simulink model "Stateflow_Eventi"  (R2023b)
settings: Solver=VariableStepAuto  StartTime=0.0  StopTime=inf  RelTol=1e-3
settings Model: Creator=sabat  LastModifiedBy=sabat
settings SolverCC: AlgebraicLoopSolver=TrustRegion
settings OptimizationCC: DefaultParameterBehavior=Inlined  EnhancedBackFolding=on  PassReuseOutputArgsAs=Individual arguments  ZeroExternalMemoryAtStartup=off  ZeroInternalMemoryAtStartup=off  OptimizeBlockOrder=speed  DifferentSizesBufferReuse=on  OptimizationCustomize=off  EfficientTunableParamExpr=on
settings DebuggingCC: ParameterTunabilityLossMsg=error
settings SFSimCC: MATLABDynamicMemAlloc=off
settings RTWCC: Description=Embedded Coder  SystemTargetFile=ert.tlc  TemplateMakefile=ert_default_tmf
settings CodeAppCC: ForceParamTrailComments=on  IgnoreCustomStorageClasses=off  OperatorAnnotations=on  SimulinkDataObjDesc=on  SFDataObjDesc=on  InsertBlockDesc=on
settings ERTTargetCC: TargetLangStandard=C99 (ISO)  GenerateSampleERTMain=on  InlinedParameterPlacement=NonHierarchical  ERTCustomFileTemplate=example_file_process.tlc

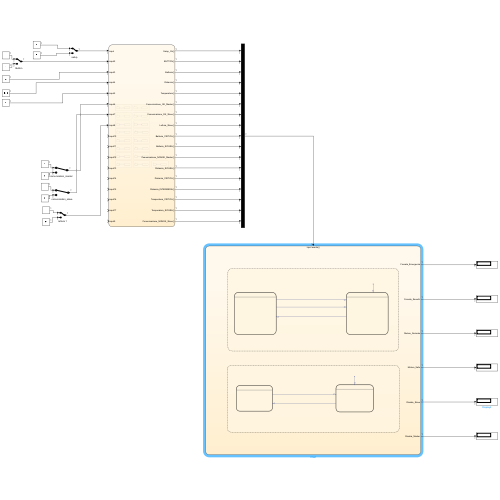
[thumbnail: Simulink's stored preview of the top-level diagram]
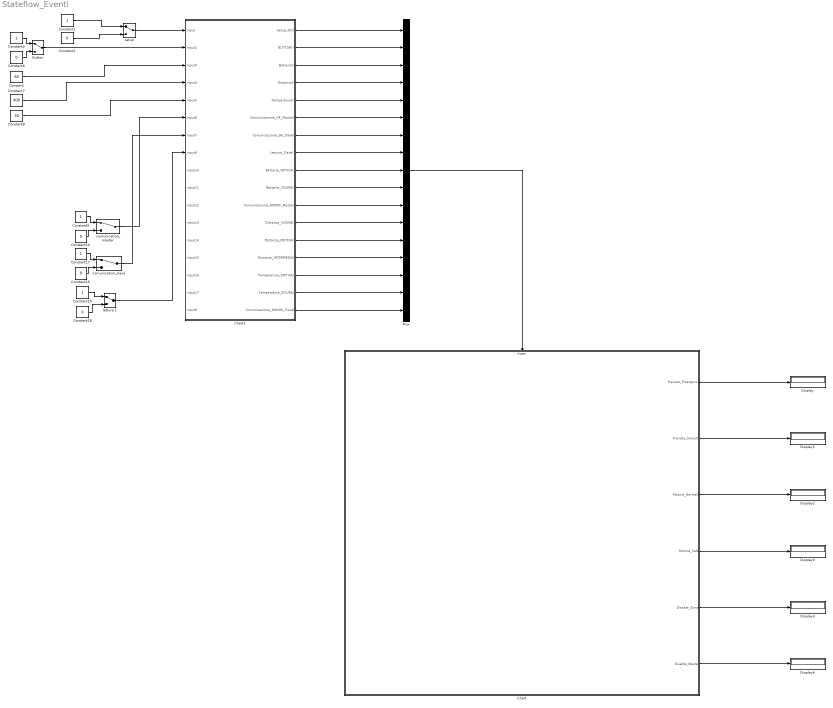
== system Stateflow_Eventi ==
  Button : ManualSwitch
  Chart : Stateflow chart  TreatAsAtomicUnit=on
  Chart3 : Stateflow chart  TreatAsAtomicUnit=on
  Constant : Constant  Value=60
  Constant{1,5,9,17,19} (5 alike) : Constant
  Constant{2,6,10,16,18} (5 alike) : Constant  Value=0
  Constant7 : Constant  Value=400
  Constant8 : Constant  Value=30
  Display{,1..4,6} (6 alike) : Display
  Mux : Mux  Inputs=17
  comunication_master : ManualSwitch
  comunication_slave : ManualSwitch
  lettura 1 : ManualSwitch
  setup : ManualSwitch
  wires:
  Constant2/1 -> setup/2
  Constant1/1 -> setup/1
  Constant6/1 -> Button/2
  Constant5/1 -> Button/1
  Button/1 -> Chart3/2(input2)
  Constant/1 -> Chart3/3(input3)
  Constant7/1 -> Chart3/4(input4)
  Constant8/1 -> Chart3/5(input5)
  comunication_master/1 -> Chart3/6(input6)
  Constant9/1 -> comunication_master/1
  Constant10/1 -> comunication_master/2
  Chart/4(Motore_Safe) -> Display3/1
  Chart/1(Frenata_Emergenza) -> Display/1
  Chart/2(Frenata_Smooth) -> Display1/1
  Chart/3(Motore_Normale) -> Display2/1
  Chart/5(Disable_Slave) -> Display4/1
  Chart/6(Disable_Master) -> Display6/1
  Constant17/1 -> comunication_slave/1
  Constant16/1 -> comunication_slave/2
  comunication_slave/1 -> Chart3/7(input7)
  Constant19/1 -> lettura 1/1
  Constant18/1 -> lettura 1/2
  lettura 1/1 -> Chart3/8(input8)
  Chart3/1(Setup_Ok()) -> Mux/1
  Chart3/2(BUTTON()) -> Mux/2
  Chart3/3(Batteria()) -> Mux/3
  Chart3/4(Distanza()) -> Mux/4
  Chart3/5(Temperatura()) -> Mux/5
  Chart3/6(Comunicazione_OK_Master()) -> Mux/6
  Chart3/7(Comunicazione_OK_Slave()) -> Mux/7
  Chart3/8(Lettura_Slave()) -> Mux/8
  Chart3/9(Batteria_CRITICA()) -> Mux/9
  Chart3/10(Batteria_SICURA()) -> Mux/10
  Chart3/11(Comunicazione_NONOK_Master()) -> Mux/11
  Chart3/12(Distanza_SICURA()) -> Mux/12
  Chart3/13(Distanza_CRITICA()) -> Mux/13
  Chart3/14(Distanza_INTERMEDIA()) -> Mux/14
  Chart3/15(Temperatura_CRITICA()) -> Mux/15
  Chart3/16(Temperatura_SICURA()) -> Mux/16
  Chart3/17(Comunicazione_NONOK_Slave()) -> Mux/17
  Mux/1 -> Chart/Trigger
  setup/1 -> Chart3/1(input)

== stateflow chart Stateflow_Eventi/Chart ==
  state MASTER [parallel]
    settings: executionOrder=1
    state Master_Acceso
      state Attuazione_Critici
        %Devo fermare il veicolo
      state Lettura_Critici_Eseguita
        %La lettura è andata a buon fine
      state Frenata_Lieve
        %Devo frenare lievemente
      state ACCESO
        %Sistema acceso
        %si sta eseguendo la setup
      state Pronto_A_Leggere_Critici
        %Devo leggere i sensori critici
      state Lettura_Non_Critici_Eseguita
        %Ho eseguito la lettura degli altri sensori
      state Attuazione_Degradata
        %Ho attuato e ora devo
        %ricominciare il ciclo
      state Attuazione
        %La comunicazione è andata
        %bene e ora posso attuare
      state Pronta_Comunicazione
        %Posso eseguire la comunicazione
      state Disabilito_Slave
        %Comunicazione andata male
        %devo disabilitare lo slave e attuare
        %di conseguenza
      Frenata_Lieve -> MASTER.Master_Acceso.ACCESO : [after(1, Distanza_SICURA)]{Frenata_Smooth = 0}
      Attuazione_Critici -> MASTER.Master_Acceso.ACCESO : [after(1, Distanza_SICURA) && after(1, Temperatura_SICURA) && after(1, Batteria_SICURA)]{Frenata_Emergenza = 0}
      Lettura_Critici_Eseguita -> Attuazione_Critici [order 1] : [after(1, Distanza_CRITICA) || after(1, Batteria_CRITICA) || after(1, Temperatura_CRITICA)]{Frenata_Emergenza =1}
      (default) -> MASTER.Master_Acceso.ACCESO
      MASTER.Master_Acceso.ACCESO -> Pronto_A_Leggere_Critici [order 1] : [after(1, Setup_Ok) ]{Disable_Slave = 0}
      Lettura_Critici_Eseguita -> Frenata_Lieve [order 3] : [after(1, Distanza_INTERMEDIA) && after(1,  Batteria_SICURA)]{Frenata_Smooth =1}
      Pronto_A_Leggere_Critici -> Lettura_Critici_Eseguita : [after(Lettura_Critici, msec) ]
      MASTER.Master_Acceso.ACCESO -> Pronto_A_Leggere_Critici [order 2] : [after(Timer_Setup_Elapsed, msec)]{Disable_Slave =1}
      Lettura_Critici_Eseguita -> Lettura_Non_Critici_Eseguita [order 2] : [after(Lettura_Non_Critici, msec)]
      Attuazione_Degradata -> MASTER.Master_Acceso.ACCESO : [after(Timeout_Ciclo,msec)]{Motore_Safe =0}
      MASTER.Master_Acceso.Attuazione -> Pronto_A_Leggere_Critici : [after(Timeout_Ciclo,msec)]{Motore_Normale =0}
      Lettura_Non_Critici_Eseguita -> Attuazione_Degradata [order 2] : [Disable_Slave == 1]{Motore_Safe = 1}
      Lettura_Non_Critici_Eseguita -> MASTER.Master_Acceso.Pronta_Comunicazione [order 1] : [Disable_Slave == 0]
      Disabilito_Slave -> Attuazione_Degradata : [Disable_Slave == 1]{Motore_Safe =1}
      MASTER.Master_Acceso.Pronta_Comunicazione -> MASTER.Master_Acceso.Attuazione [order 1] : [after(1, Comunicazione_OK_Master)]{Motore_Normale =1}
      MASTER.Master_Acceso.Pronta_Comunicazione -> Disabilito_Slave [order 2] : [after(1, Comunicazione_NONOK_Master)]{Disable_Slave =1}
    state Master_Spento
      state SPENTO
        %Sistema non alimentato
      (default) -> MASTER.Master_Spento.SPENTO
    (default) -> Master_Spento
    Master_Acceso -> Master_Spento : [BUTTON == 0 ]
    Master_Spento -> Master_Acceso : [BUTTON == 1 && Disable_Master ==0]
  state SLAVE [parallel]
    settings: executionOrder=2
    state Slave_Spento
      state SPENTO
        %Sistema non alimentato
      (default) -> SLAVE.Slave_Spento.SPENTO
    state Slave_Acceso
      state Spento_Master
        %Devo fermare il veicolo
        % e spegnere il master
      state Pronta_Comunicazione
        %Posso eseguire la comunicazione
      state Pronto_A_Leggere
        %Devo leggere i sensori
      state ACCESO
        %Sistema acceso
        %si sta eseguendo la setup
      state Attuazione
        %La comunicazione è andata
        %bene e ora posso attuare
      Spento_Master -> SLAVE.Slave_Acceso.ACCESO : [after(Time_For_Recovery, msec)]{Disable_Master = 0}
      SLAVE.Slave_Acceso.Pronta_Comunicazione -> Spento_Master [order 2] : [after(1, Comunicazione_NONOK_Slave)]{Disable_Master = 1}
      (default) -> SLAVE.Slave_Acceso.ACCESO
      SLAVE.Slave_Acceso.ACCESO -> Pronto_A_Leggere : [after(1, Setup_Ok)]
      Pronto_A_Leggere -> SLAVE.Slave_Acceso.Pronta_Comunicazione [order 1] : [after(1, Lettura_Slave)]
      Pronto_A_Leggere -> SLAVE.Slave_Acceso.ACCESO [order 2] : [Frenata_Emergenza == 1]
      SLAVE.Slave_Acceso.Attuazione -> Pronto_A_Leggere [order 1] : [after(Timeout_Ciclo,msec)]
      SLAVE.Slave_Acceso.Pronta_Comunicazione -> SLAVE.Slave_Acceso.ACCESO [order 3] : [Frenata_Emergenza == 1 ]
      SLAVE.Slave_Acceso.Attuazione -> SLAVE.Slave_Acceso.ACCESO [order 2] : [Frenata_Emergenza == 1]
      SLAVE.Slave_Acceso.Pronta_Comunicazione -> SLAVE.Slave_Acceso.Attuazione [order 1] : [after(1, Comunicazione_OK_Slave)]
    (default) -> Slave_Spento
    Slave_Acceso -> Slave_Spento : [BUTTON == 0 ]
    Slave_Spento -> Slave_Acceso : [BUTTON == 1 && Disable_Slave ==0]
  data: Frenata_Emergenza output double; Frenata_Smooth output double; Motore_Normale output double; Motore_Safe output double; Disable_Slave output double =0; Disable_Master output double =0; Lettura_Critici local =10; Lettura_Non_Critici local =10; Timer_Setup_Elapsed local =10; Timeout_Ciclo local =10; Time_For_Recovery local =10
  events: Setup_Ok input FUNCTION_CALL_EVENT; BUTTON input FUNCTION_CALL_EVENT; Batteria input FUNCTION_CALL_EVENT; Distanza input FUNCTION_CALL_EVENT; Temperatura input FUNCTION_CALL_EVENT; Comunicazione_OK_Master input RISING_EDGE_EVENT; Comunicazione_OK_Slave input FUNCTION_CALL_EVENT; Lettura_Slave input FUNCTION_CALL_EVENT; Batteria_CRITICA input RISING_EDGE_EVENT; Batteria_SICURA input RISING_EDGE_EVENT; Comunicazione_NONOK_Master input RISING_EDGE_EVENT; Distanza_SICURA input RISING_EDGE_EVENT; Distanza_CRITICA input RISING_EDGE_EVENT; Distanza_INTERMEDIA input RISING_EDGE_EVENT; Temperatura_CRITICA input RISING_EDGE_EVENT; Temperatura_SICURA input RISING_EDGE_EVENT; Comunicazione_NONOK_Slave input RISING_EDGE_EVENT

== stateflow chart Stateflow_Eventi/Chart3 ==
  state Input [parallel]
    settings: executionOrder=1
    state off
    state on
    (default) -> Input.off
    Input.off -> Input.on : [input == 1]{send(Setup_Ok);}
    Input.on -> Input.off : [input == 0]
  state Input3 [parallel]
    settings: executionOrder=3
    state off
    state on
    (default) -> Input3.off
    Input3.off -> Input3.on : [input3 == 1]{send(Batteria);}
    Input3.on -> Input3.off : [input3 == 0]
  state Input2 [parallel]
    settings: executionOrder=2
    state off
    state on
    (default) -> Input2.off
    Input2.off -> Input2.on : [input2 == 1]{send(BUTTON);}
    Input2.on -> Input2.off : [input2 == 0]
  state Input4 [parallel]
    settings: executionOrder=4
    state off
    state on
    (default) -> Input4.off
    Input4.off -> Input4.on : [input4 == 1]{send(Distanza);}
    Input4.on -> Input4.off : [input4 == 0]
  state Input6 [parallel]
    settings: executionOrder=6
    state off
    state on
    (default) -> Input6.off
    Input6.off -> Input6.on : [input6 == 1]{send(Comunicazione_OK_Master);}
    Input6.on -> Input6.off : [input6 == 0]
  state Input5 [parallel]
    settings: executionOrder=5
    state off
    state on
    (default) -> Input5.off
    Input5.off -> Input5.on : [input5 == 1]{send(Temperatura);}
    Input5.on -> Input5.off : [input5 == 0]
  state Input7 [parallel]
    settings: executionOrder=7
    state off
    state on
    (default) -> Input7.off
    Input7.off -> Input7.on : [input7 == 1]{send(Comunicazione_OK_Slave);}
    Input7.on -> Input7.off : [input7 == 0]
  state Input8 [parallel]
    settings: executionOrder=8
    state off
    state on
    (default) -> Input8.off
    Input8.off -> Input8.on : [input8 == 1]{send(Lettura_Slave);}
    Input8.on -> Input8.off : [input8 == 0]
  state Input9 [parallel]
    settings: executionOrder=9
    state off
    state on
    (default) -> Input9.off
    Input9.off -> Input9.on : [input9 == 1]{send(Batteria_CRITICA);}
    Input9.on -> Input9.off : [input9 == 0]
  state Input10 [parallel]
    settings: executionOrder=10
    state off
    state on
    (default) -> Input10.off
    Input10.off -> Input10.on : [input10 == 1]{send(Batteria_SICURA);}
    Input10.on -> Input10.off : [input10 == 0]
  state Input11 [parallel]
    settings: executionOrder=11
    state off
    state on
    (default) -> Input11.off
    Input11.off -> Input11.on : [input11 == 1]{send(Comunicazione_NONOK_Master);}
    Input11.on -> Input11.off : [input11 == 0]
  state Input12 [parallel]
    settings: executionOrder=12
    state off
    state on
    (default) -> Input12.off
    Input12.off -> Input12.on : [input12 == 1]{send(Distanza_SICURA);}
    Input12.on -> Input12.off : [input12 == 0]
  state Input13 [parallel]
    settings: executionOrder=13
    state off
    state on
    (default) -> Input13.off
    Input13.off -> Input13.on : [input13 == 1]{send(Distanza_CRITICA);}
    Input13.on -> Input13.off : [input13 == 0]
  state Input14 [parallel]
    settings: executionOrder=14
    state off
    state on
    (default) -> Input14.off
    Input14.off -> Input14.on : [input14 == 1]{send(Distanza_INTERMEDIA);}
    Input14.on -> Input14.off : [input14 == 0]
  state Input15 [parallel]
    settings: executionOrder=15
    state off
    state on
    (default) -> Input15.off
    Input15.off -> Input15.on : [input15 == 1]{send(Temperatura_CRITICA);}
    Input15.on -> Input15.off : [input15 == 0]
  state Input16 [parallel]
    settings: executionOrder=16
    state off
    state on
    (default) -> Input16.off
    Input16.off -> Input16.on : [input16 == 1]{send(Temperatura_SICURA);}
    Input16.on -> Input16.off : [input16 == 0]
  state Input17 [parallel]
    settings: executionOrder=17
    state off
    state on
    (default) -> Input17.off
    Input17.off -> Input17.on : [input17 == 1]{send(Comunicazione_NONOK_Slave);}
    Input17.on -> Input17.off : [input17 == 0]
  data: input input; input2 input; input3 input; input4 input; input5 input; input6 input; input7 input; input8 input; input10 input; input11 input; input12 input; input13 input; input14 input; input15 input; input16 input; input17 input; input9 input
  events: Setup_Ok output FUNCTION_CALL_EVENT; BUTTON output FUNCTION_CALL_EVENT; Batteria output FUNCTION_CALL_EVENT; Distanza output FUNCTION_CALL_EVENT; Temperatura output FUNCTION_CALL_EVENT; Comunicazione_OK_Master output FUNCTION_CALL_EVENT; Comunicazione_OK_Slave output FUNCTION_CALL_EVENT; Lettura_Slave output FUNCTION_CALL_EVENT; Batteria_CRITICA output FUNCTION_CALL_EVENT; Batteria_SICURA output FUNCTION_CALL_EVENT; Comunicazione_NONOK_Master output FUNCTION_CALL_EVENT; Distanza_SICURA output FUNCTION_CALL_EVENT; Distanza_CRITICA output FUNCTION_CALL_EVENT; Distanza_INTERMEDIA output FUNCTION_CALL_EVENT; Temperatura_CRITICA output FUNCTION_CALL_EVENT; Temperatura_SICURA output FUNCTION_CALL_EVENT; Comunicazione_NONOK_Slave output FUNCTION_CALL_EVENT
